simulink model "sampleModel1851"  (R2023a)
settings: Solver=VariableStepAuto  StartTime=0.0  StopTime=10.0  RelTol=1e-3
libraries: simulink x3, hdlsllib x3
settings Model: Creator=user1  LastModifiedBy=user1

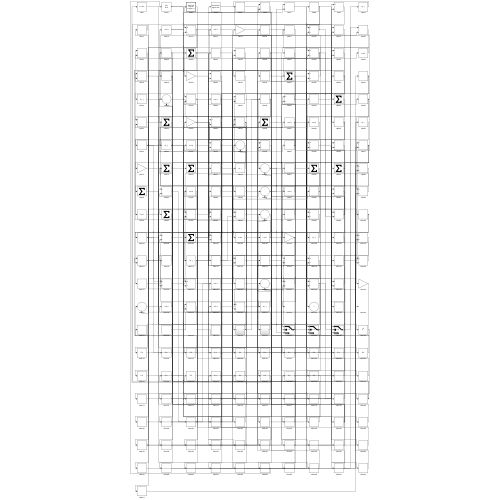
[thumbnail: Simulink's stored preview of the top-level diagram]
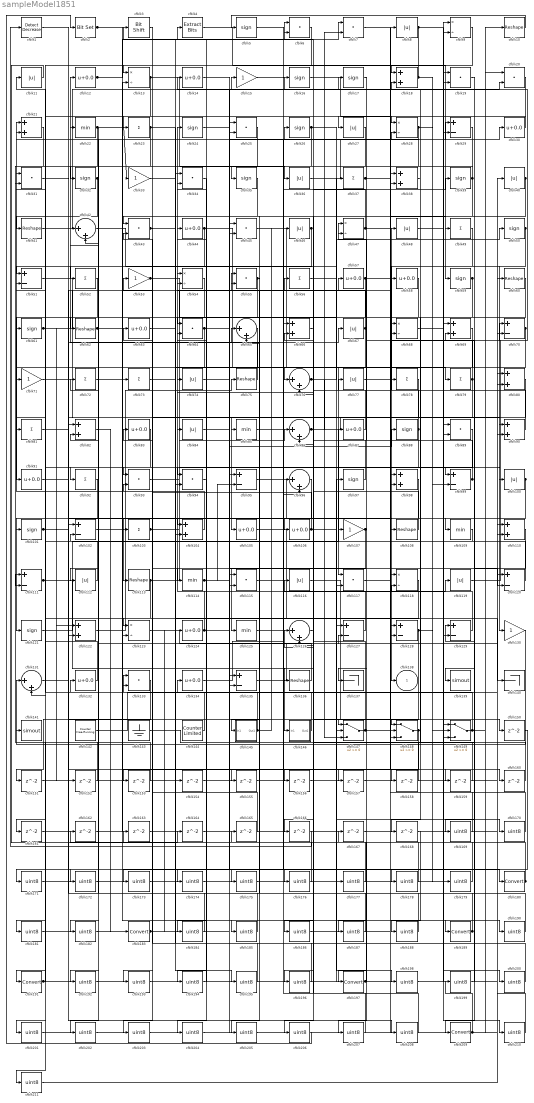
== system sampleModel1851 ==
  cfblk1 : simulink/Logic and Bit Operations/Detect Decrease  vinit=0.0  OutDataTypeStr=boolean
      settings: LibrarySourceBlock=|
      | hdlsllib/Logic and Bit
      | Operations/Detect
      | Decrease
  cfblk{10,41,60,62,75,108,113,136} (8 alike) : Reshape
  cfblk{8,11,27,36,40,46,48,67,74,77,84,100,112,116,119} (15 alike) : Abs  SaturateOnIntegerOverflow=off
  cfblk{5,16..17,24,26,32,35,39,50,59,61,88,97,101,121} (15 alike) : Signum
  cfblk{29,51,70,95,99,102,111,120,127..129,135} (12 alike) : Sum  Inputs=+-
  cfblk{23,37,49,52,56,72..73,78..79,81,92,103} (12 alike) : Sum  Inputs=+
  cfblk{18,21,38,66,69,80,82,90,98,104,110,122} (12 alike) : Sum
  cfblk{12,14,30,44,57..58,63,83,87,91,105..106,124,132,134} (15 alike) : Bias  Bias=0.0  SaturateOnIntegerOverflow=off
  cfblk{15,33,53,71,107,130} (6 alike) : Gain
  cfblk{22,85,109,114,125} (5 alike) : MinMax
  cfblk{6..7,19..20,25,31,34,43,45,55,64,89,93..94,115,117,133} (17 alike) : DotProduct  OutDataTypeStr=Inherit: Inherit via internal rule
  cfblk{9,13,28,47,54,68,118,123} (8 alike) : Product  Inputs=*/  RndMeth=Zero  SaturateOnIntegerOverflow=on
  cfblk{42,65,76,86,96,126,131} (7 alike) : Sum  Inputs=|++
  cfblk137 : Terminator
  cfblk139 : ToWorkspace  VariableName=simout  SaveFormat=Timeseries  SampleTime=-1
  cfblk140 : Terminator
  cfblk141 : ToWorkspace  VariableName=simout  SaveFormat=Timeseries  SampleTime=-1
  cfblk142 : hdlsllib/Sources/Counter Free-Running  NumBits=16  tsamp=-1
  cfblk143 : Ground
  cfblk144 : hdlsllib/Sources/Counter Limited  uplimit=7  tsamp=-1
  cfblk145 : Subsystem
      settings: LibrarySourceBlock=|
      | hdlsllib/Ports &
      | Subsystems/Subsystem
  cfblk146 : Subsystem
      settings: LibrarySourceBlock=|
      | hdlsllib/Ports &
      | Subsystems/Subsystem
  cfblk147 : Switch  SaturateOnIntegerOverflow=off  InputSameDT=off
  cfblk148 : Switch  SaturateOnIntegerOverflow=off  InputSameDT=off
  cfblk149 : Switch  SaturateOnIntegerOverflow=off  InputSameDT=off
  cfblk{150..168} (19 alike) : Delay  SampleTime=1
  cfblk{169..179,181..182,184..188,190,192..196,198..208,210..211} (37 alike) : DataTypeConversion  OutDataTypeStr=uint8  SaturateOnIntegerOverflow=off  RndMeth=Floor
  cfblk{180,183,189,191,197,209} (6 alike) : DataTypeConversion  SaturateOnIntegerOverflow=off  RndMeth=Floor
  cfblk2 : simulink/Logic and Bit Operations/Bit Set  iBit=0
      settings: LibrarySourceBlock=|
      | hdlsllib/Logic and Bit
      | Operations/Bit Set
  cfblk3 : hdlsllib/Logic and Bit Operations/Bit Shift  mode=Shift Left Logical  N=0
  cfblk4 : simulink/Logic and Bit Operations/Extract Bits  bitsToExtract=Upper half  numBits=8  bitIdxRange=[0 7]  outScalingMode=Preserve fixed-point scaling
      settings: LibrarySourceBlock=|
      | hdlsllib/Logic and Bit
      | Operations/Extract Bits
  cfblk138 : Outport  VectorParamsAs1DForOutWhenUnconnected=off
  wires:
  cfblk122/1 -> cfblk75/1
  cfblk104/1 -> cfblk21/1
  cfblk149/1 -> cfblk133/1, cfblk10/1
  cfblk119/1 -> cfblk15/1
  cfblk51/1 -> cfblk105/1
  cfblk103/1 -> cfblk57/1, cfblk106/1
  cfblk28/1 -> cfblk21/2, cfblk94/2, cfblk99/2
  cfblk13/1 -> cfblk35/1, cfblk71/1
  cfblk45/1 -> cfblk79/1
  cfblk129/1 -> cfblk24/1
  cfblk23/1 -> cfblk76/1, cfblk122/2, cfblk160/1
  cfblk55/1 -> cfblk64/1, cfblk205/1
  cfblk124/1 -> cfblk84/1, cfblk88/1
  cfblk38/1 -> cfblk27/1
  cfblk113/1 -> cfblk86/1, cfblk58/1, cfblk181/1
  cfblk50/1 -> cfblk130/1, cfblk148/3
  cfblk116/1 -> cfblk148/1
  cfblk110/1 -> cfblk209/1
  cfblk100/1 -> cfblk121/1, cfblk147/2
  cfblk32/1 -> cfblk92/1, cfblk81/1
  cfblk37/1 -> cfblk137/1, cfblk159/1
  cfblk99/1 -> cfblk47/1, cfblk6/2
  cfblk40/1 -> cfblk43/1, cfblk166/1
  cfblk101/1 -> cfblk147/1, cfblk152/1
  cfblk49/1 -> cfblk138/1
  cfblk4/1 -> cfblk59/1
  cfblk143/1 -> cfblk129/1
  cfblk115/1 -> cfblk180/1
  cfblk30/1 -> cfblk28/1
  cfblk93/1 -> cfblk100/1
  cfblk44/1 -> cfblk117/1, cfblk123/2
  cfblk26/1 -> cfblk135/2, cfblk170/1
  cfblk61/1 -> cfblk56/1, cfblk122/1, cfblk208/1
  cfblk147/1 -> cfblk118/1, cfblk14/1
  cfblk75/1 -> cfblk12/1
  cfblk18/1 -> cfblk13/1, cfblk179/1
  cfblk107/1 -> cfblk125/1, cfblk193/1
  cfblk95/1 -> cfblk108/1
  cfblk79/1 -> cfblk47/2, cfblk155/1
  cfblk70/1 -> cfblk139/1, cfblk109/1, cfblk136/1
  cfblk145/1(Out1) -> cfblk83/1, cfblk46/1
  cfblk22/1 -> cfblk33/1, cfblk61/1, cfblk182/1
  cfblk64/1 -> cfblk161/1, cfblk176/1
  cfblk146/1(Out1) -> cfblk4/1
  cfblk53/1 -> cfblk127/1, cfblk95/1
  cfblk36/1 -> cfblk28/2
  cfblk148/1 -> cfblk118/2, cfblk173/1
  cfblk114/1 -> cfblk44/1, cfblk95/2, cfblk20/2
  cfblk72/1 -> cfblk189/1
  cfblk130/1 -> cfblk131/1
  cfblk111/1 -> cfblk146/1(In1), cfblk54/1
  cfblk102/1 -> cfblk113/1
  cfblk125/1 -> cfblk119/1
  cfblk16/1 -> cfblk98/1
  cfblk131/1 -> cfblk67/1
  cfblk77/1 -> cfblk48/1
  cfblk117/1 -> cfblk70/1
  cfblk9/1 -> cfblk18/1
  cfblk69/1 -> cfblk197/1
  cfblk83/1 -> cfblk131/2
  cfblk62/1 -> cfblk185/1, cfblk190/1
  cfblk67/1 -> cfblk26/1, cfblk62/1, cfblk112/1
  cfblk87/1 -> cfblk77/1
  cfblk134/1 -> cfblk39/1
  cfblk92/1 -> cfblk101/1
  cfblk7/1 -> cfblk128/1
  cfblk86/1 -> cfblk90/1, cfblk7/2
  cfblk120/1 -> cfblk55/1
  cfblk46/1 -> cfblk201/1, cfblk211/1
  cfblk41/1 -> cfblk17/1
  cfblk85/1 -> cfblk29/1
  cfblk12/1 -> cfblk73/1, cfblk6/1
  cfblk135/1 -> cfblk120/1
  cfblk132/1 -> cfblk11/1
  cfblk142/1 -> cfblk60/1
  cfblk128/1 -> cfblk149/2, cfblk196/1
  cfblk112/1 -> cfblk31/1
  cfblk2/1 -> cfblk104/2, cfblk156/1
  cfblk48/1 -> cfblk9/1
  cfblk1/1 -> cfblk85/1
  cfblk109/1 -> cfblk102/2
  cfblk82/1 -> cfblk183/1
  cfblk10/1 -> cfblk5/1
  cfblk21/1 -> cfblk31/2
  cfblk71/1 -> cfblk128/2
  cfblk84/1 -> cfblk120/2
  cfblk88/1 -> cfblk94/1, cfblk54/2
  cfblk96/1 -> cfblk191/1
  cfblk136/1 -> cfblk22/1
  cfblk123/1 -> cfblk127/2
  cfblk90/1 -> cfblk78/1
  cfblk76/1 -> cfblk37/1, cfblk147/3
  cfblk6/1 -> cfblk41/1
  cfblk14/1 -> cfblk36/1
  cfblk127/1 -> cfblk65/1
  cfblk58/1 -> cfblk148/2
  cfblk33/1 -> cfblk129/2
  cfblk105/1 -> cfblk140/1
  cfblk121/1 -> cfblk87/1
  cfblk35/1 -> cfblk114/1
  cfblk3/1 -> cfblk23/1
  cfblk25/1 -> cfblk111/2
  cfblk97/1 -> cfblk3/1
  cfblk27/1 -> cfblk52/1
  cfblk39/1 -> cfblk104/1, cfblk65/2, cfblk32/1
  cfblk47/1 -> cfblk49/1, cfblk16/1
  cfblk65/1 -> cfblk133/2
  cfblk59/1 -> cfblk103/1, cfblk168/1
  cfblk108/1 -> cfblk74/1
  cfblk20/1 -> cfblk51/1
  cfblk144/1 -> cfblk51/2
  cfblk74/1 -> cfblk30/1
  cfblk52/1 -> cfblk91/1
  cfblk43/1 -> cfblk7/1, cfblk123/1
  cfblk56/1 -> cfblk50/1
  cfblk57/1 -> cfblk145/1(In1), cfblk99/1
  cfblk8/1 -> cfblk93/1, cfblk98/2, cfblk210/1
  cfblk91/1 -> cfblk107/1
  cfblk24/1 -> cfblk135/1
  cfblk106/1 -> cfblk53/1, cfblk198/1
  cfblk31/1 -> cfblk150/1
  cfblk133/1 -> cfblk151/1
  cfblk151/1 -> cfblk70/2
  cfblk152/1 -> cfblk111/1
  cfblk118/1 -> cfblk153/1
  cfblk153/1 -> cfblk102/1
  cfblk63/1 -> cfblk154/1
  cfblk154/1 -> cfblk45/2
  cfblk155/1 -> cfblk38/2
  cfblk156/1 -> cfblk117/2
  cfblk81/1 -> cfblk157/1
  cfblk157/1 -> cfblk9/2
  cfblk5/1 -> cfblk158/1
  cfblk158/1 -> cfblk86/2
  cfblk159/1 -> cfblk76/2
  cfblk160/1 -> cfblk18/2
  cfblk161/1 -> cfblk13/2
  cfblk163/1 -> cfblk25/1
  cfblk11/1 -> cfblk164/1
  cfblk164/1 -> cfblk29/2
  cfblk165/1 -> cfblk93/2
  cfblk166/1 -> cfblk1/1
  cfblk167/1 -> cfblk90/2
  cfblk19/1 -> cfblk169/1
  cfblk169/1 -> cfblk38/1
  cfblk170/1 -> cfblk19/1
  cfblk150/1 -> cfblk171/1
  cfblk171/1 -> cfblk19/2
  cfblk89/1 -> cfblk172/1
  cfblk172/1 -> cfblk25/2
  cfblk173/1 -> cfblk89/1
  cfblk78/1 -> cfblk174/1
  cfblk174/1 -> cfblk89/2
  cfblk162/1 -> cfblk175/1
  cfblk175/1 -> cfblk55/2
  cfblk176/1 -> cfblk162/1
  cfblk42/1 -> cfblk177/1
  cfblk177/1 -> cfblk43/2
  cfblk15/1 -> cfblk178/1
  cfblk178/1 -> cfblk42/1
  cfblk179/1 -> cfblk42/2
  cfblk180/1 -> cfblk116/1, cfblk64/2
  cfblk181/1 -> cfblk115/1
  cfblk182/1 -> cfblk115/2
  cfblk183/1 -> cfblk163/1, cfblk124/1
  cfblk60/1 -> cfblk184/1
  cfblk184/1 -> cfblk82/1
  cfblk185/1 -> cfblk82/2
  cfblk126/1 -> cfblk186/1
  cfblk186/1 -> cfblk8/1
  cfblk29/1 -> cfblk187/1
  cfblk187/1 -> cfblk126/1
  cfblk168/1 -> cfblk188/1
  cfblk188/1 -> cfblk126/2
  cfblk189/1 -> cfblk165/1, cfblk149/1, cfblk132/1
  cfblk190/1 -> cfblk72/1
  cfblk191/1 -> cfblk97/1, cfblk149/3, cfblk141/1
  cfblk54/1 -> cfblk192/1
  cfblk192/1 -> cfblk96/1
  cfblk193/1 -> cfblk96/2
  cfblk34/1 -> cfblk194/1
  cfblk194/1 -> cfblk134/1
  cfblk73/1 -> cfblk195/1
  cfblk195/1 -> cfblk34/1
  cfblk196/1 -> cfblk34/2
  cfblk197/1 -> cfblk167/1, cfblk40/1
  cfblk198/1 -> cfblk69/1
  cfblk199/1 -> cfblk69/2
  cfblk68/1 -> cfblk200/1
  cfblk200/1 -> cfblk63/1
  cfblk201/1 -> cfblk68/1
  cfblk98/1 -> cfblk202/1
  cfblk202/1 -> cfblk68/2
  cfblk80/1 -> cfblk203/1
  cfblk203/1 -> cfblk45/1
  cfblk94/1 -> cfblk204/1
  cfblk204/1 -> cfblk80/1
  cfblk205/1 -> cfblk80/2
  cfblk66/1 -> cfblk206/1
  cfblk206/1 -> cfblk2/1
  cfblk17/1 -> cfblk207/1
  cfblk207/1 -> cfblk66/1
  cfblk208/1 -> cfblk66/2
  cfblk209/1 -> cfblk199/1, cfblk20/1
  cfblk210/1 -> cfblk110/1
  cfblk211/1 -> cfblk110/2

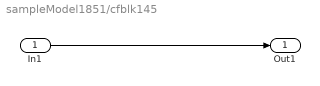
== system sampleModel1851/cfblk145 ==
  In1 : Inport
  Out1 : Outport
  wires:
  In1/1 -> Out1/1

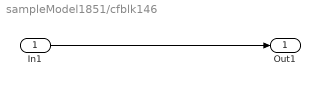
== system sampleModel1851/cfblk146 ==
  In1 : Inport
  Out1 : Outport
  wires:
  In1/1 -> Out1/1
